simulink model "State_Space_Model"  (R2025b)
settings: Solver=VariableStepAuto  StartTime=0.0  StopTime=10.0  RelTol=1e-3
settings Model: Creator=CAM  LastModifiedBy=CAM

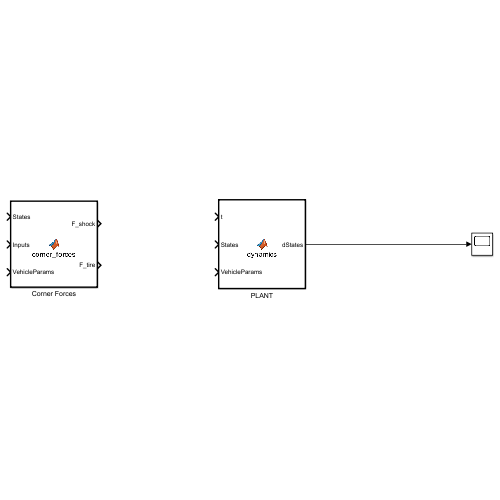
[thumbnail: Simulink's stored preview of the top-level diagram]
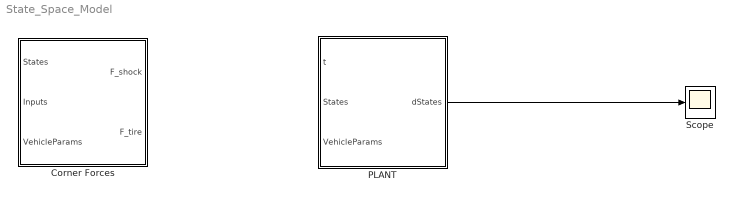
== system State_Space_Model ==
  Corner Forces : MATLAB Function  TreatAsAtomicUnit=on
  PLANT : MATLAB Function  TreatAsAtomicUnit=on
  Scope : Scope
  wires:
  PLANT/1(dStates) -> Scope/1

== matlab function State_Space_Model/PLANT ==
  data: t input; dStates output; States input; VehicleParams input
function dStates = dynamics(t, States, VehicleParams)

    % 1. Get Inputs (Road & Driver)
    Inputs = get_road_profile(t, VehicleParams.speed);
    [Ax_g, Ay_g] = get_driver_inputs(t);
    
    % 2. Call Block A (Get Forces)
    [F_sus, F_tire] = calculate_forces(States, Inputs, VehicleParams);
    
    % 3. Solve Equations of Motion (F=ma)
    Ms = VehicleParams.Ms;
    Ixx = VehicleParams.Ixx;
    Iyy = VehicleParams.Iyy;
    
    % Sum of forces for Body Z
    Zs_2dot = sum(F_sus) / Ms;
    
    % Sum of Moments for Body Theta (Pitch)
    % (Remember to add Inertial moments M_pitch = Ms*Ax*h here)
    M_pitch_inertial = -Ms * (Ax_g*9.81) * VehicleParams.h;
    Sum_Moment_Y = (F_sus(3)+F_sus(4))*VehicleParams.b - ...
                   (F_sus(1)+F_sus(2))*VehicleParams.a + M_pitch_inertial;
    theta_2dot = Sum_Moment_Y / Iyy;
    
    % Sum of Moments for Body Phi (Roll)
    % ... (Similar logic for Roll)
    
    % Wheel Accelerations
    Zu_2dot = (F_tire - F_sus) ./ VehicleParams.m_unsprung;
    
    % 4. Pack Derivatives
    dStates = [States(8:14); Zs_2dot; theta_2dot; ... ; Zu_2dot];
 end

== matlab function State_Space_Model/Corner Forces ==
  data: States input; Inputs input; F_shock output; F_tire output; VehicleParams input
function [F_shock, F_tire]  = corner_forces(States, Inputs, VehicleParams)

    % Unpack States
    Zs = States(1); theta = States(2); phi = States(3);
    Zu = States(4:7); % [Zu1, Zu2, Zu3, Zu4]
    
    Zs_dot = States(8); theta_dot = States(9); phi_dot = States(10);
    Zu_dot = States(11:14);
    
    % Unpack Inputs
    Zg = Inputs.Zg; % Road height at 4 corners
    
    % Geometry (Local calc or passed in params)
    a = VehicleParams.a; b = VehicleParams.b;
    w_f = VehicleParams.w_f; w_r = VehicleParams.w_r;
    
    % 1. Calculate Deflections (Suspension Travel)
    % Position of body at each corner mount point
    Z_body_mount = zeros(4,1);
    Z_body_mount(1) = Zs - a*theta - w_f*phi; % FL
    Z_body_mount(2) = Zs - a*theta + w_f*phi; % FR
    Z_body_mount(3) = Zs + b*theta - w_r*phi; % RL
    Z_body_mount(4) = Zs + b*theta + w_r*phi; % RR
    
    suspension_deflection = Z_body_mount - Zu;
    suspension_velocity   = ... % (Similar derivative math)
    
    % 2. Calculate Forces (F = kx + cv)
    F_k = VehicleParams.k_sus .* suspension_deflection;
    F_c   = VehicleParams.c_sus .* suspension_velocity;
    
    F_shock = F_k + F_c;
    
    % 3. Tire Forces
    F_tire = VehicleParams.kt .* (Zg - Zu);
end
